simulink model "OBCSystem"  (R2025b)
settings: Solver=FixedStepAuto  StartTime=0.0  StopTime=100e-3  RelTol=1e-3  EnableMultiTasking=on
PreLoadFcn:
  | %% Load OBCSystem initialization parameters
  | initScriptPath = fullfile(fileparts(which('OBCSystem')), '..', 'SupportFiles', 'Scripts', 'OBCSystem_init.m');
  | if isfile(initScriptPath)
  |     evalin('base', fileread(initScriptPath));
  | else
  |     warning('OBCSystem:initNotFound', 'OBCSystem_init.m not found at: %s', initScriptPath);
  | end
InitFcn:
  | mode = str2double(get_param('OBCSystem/System/SimulationMode','value'));
  | enableLogging = str2double(get_param('OBCSystem/System/On-Board Charger/HIL/EnableHighResLogging','value'));
  | 
  | % If the charger runs on the FPGA AND high-resolution logging is enabled,
  | % uncomment interrupt setup. Comment otherwise
  | if ((mode == 2) && (enableLogging == 1))
  |     set_param('OBCSystem/Interrupt Setup','Commented','off');
  | else
  |     set_param('OBCSystem/Interrupt Setup','Commented','on');
  | end
  | 
  | % If DMA streaming is enambled and simulation time exceeds 30s, then throw an error
  | maxStopTime = 30;   % seconds
  | stopTimeStr = get_param(bdroot, 'StopTime');
  | stopTimeVal = str2double(stopTimeStr);
  | 
  | if enableLogging && stopTimeVal > maxStopTime
  |     error('DMA streaming is enabled, but StopTime = %.3f s exceeds the allowed %.3f s.', ...
  |           stopTimeVal, maxStopTime);
  | end
undefined symbols (not defined in the file): DAB, DAB_CCCV_Ki, DAB_CCCV_Kp, DAB_CCCV_Kt, DAB_Charging, DAB_CurrentReference, DAB_DCOffset, DAB_PhaseShift_LowerSat, DAB_PhaseShift_UpperSat, DAB_PhaseShiftInit, DAB_PhaseToDeg, DAB_PID_Kd, DAB_PID_Ki, DAB_PID_Kp, DAB_PID_LowerSat, DAB_PID_N, DAB_PID_UpperSat, Fourier_class, FPGA, FrameSize, getfullname, grid, Instr_EffGain, Instr_PinGain, Instr_PoutGain, Instr_pUtoDeg, Instr_RippleGain, Instr_SoCGain, IO334, Ki_current, Ki_voltage, Kp_current, Kp_voltage, MIL_or_HIL, OBC_template1, OpenLoopDuty, OpenLoopEnable, PCIe_RT, PFC_Current_Kb, PFC_Current_LowerSat, PFC_Current_UpperSat, PFC_Sat_DC_Lower, PFC_Sat_DC_Upper, PFC_Sat_iL_Lower, PFC_Sat_iL_Upper, PFC_Sat_Pwr_Lower, PFC_Sat_Pwr_Upper, PFC_Voltage_Kb, PFC_Voltage_LowerSat, PFC_Voltage_UpperSat, Rblock, Real, Time, totemPole, ts_CPU, ts_FPGA_clk, ts_FPGA_mdl, VectorSize
libraries: nesl_utility x27, fl_lib x24, speedgoatlib_hdlCoder_IO3xx x20, ee_lib x12, simulink x4, eeGeneralControl x4, slpidlib x3, pwm_cpulib x2, batteryecm_lib x2, slrealtimeloglib x2, pwm_fpgalib x2, speedgoatlib_interrupt x1
(part 2 of 4)

== system OBCSystem/User Interface/Instrumentation/Fourier1 ==
  In : Inport
  Fourier Analysis : eeGeneralControl/Fourier Analysis  f=50  n=2  M0=Fourier_class([0 0]).objParamMappingDerived.NewDerivedParam.M0  Ph0=Fourier_class([0 0]).objParamMappingDerived.NewDerivedParam.Ph0  BufferSize=8192  Ts=ts_CPU
  Gain : Gain  Gain=180/pi
  Mag : Outport  VectorParamsAs1DForOutWhenUnconnected=off
  Phase : Outport  Port=2  VectorParamsAs1DForOutWhenUnconnected=off
  wires:
  Gain/1 -> Phase/1
  Fourier Analysis/2 -> Gain/1
  Fourier Analysis/1 -> Mag/1
  In/1 -> Fourier Analysis/1

== system OBCSystem/User Interface/Instrumentation/Mean1 ==
  In : Inport
  Moving Average : eeGeneralControl/Moving Average  VariantControl=Variant1  LabelModeActiveChoice=Discrete  f=Instr_MeanFreq  x0=0  BufferSize=8192  Ts=ts_CPU
  Mean : Outport  VectorParamsAs1DForOutWhenUnconnected=off
  wires:
  Moving Average/1 -> Mean/1
  In/1 -> Moving Average/1

== system OBCSystem/User Interface/Instrumentation/Mean2 ==
  In : Inport
  Moving Average : eeGeneralControl/Moving Average  VariantControl=Variant1  LabelModeActiveChoice=Discrete  f=Instr_MeanFreq  x0=0  BufferSize=8192  Ts=ts_CPU
  Mean : Outport  VectorParamsAs1DForOutWhenUnconnected=off
  wires:
  Moving Average/1 -> Mean/1
  In/1 -> Moving Average/1

== system OBCSystem/User Interface/Instrumentation/THD ==
  In : Inport
  Gain : Gain  Gain=1/100  SampleTime=ts_CPU
  Total Harmonic Distortion : eeTotalHarmonicDistorsion/Total Harmonic Distortion  f=50  Ts=ts_CPU
  THD : Outport  VectorParamsAs1DForOutWhenUnconnected=off
  wires:
  Gain/1 -> THD/1
  In/1 -> Total Harmonic Distortion/1
  Total Harmonic Distortion/1 -> Gain/1

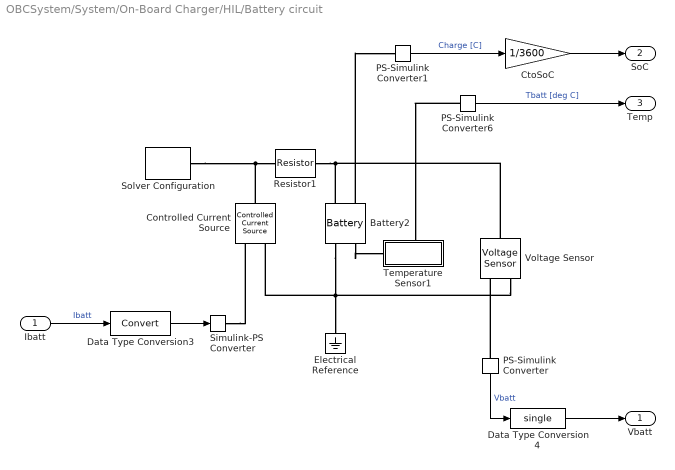
== system OBCSystem/System/On-Board Charger/HIL/Battery circuit ==
  Ibatt : Inport
  Battery2 : batteryecm_lib/Battery  Vnom=Battery_Vnom V  prm_dir=simscape.enum.battery.prm_dir.disabled  R1_dis=2 Ohm  R1_ch=2 Ohm  R1=Battery_R1 Ohm  prm_AH=simscape.enum.battery.prm_AH.finite  AH=Battery_AH A*hr  V1=Battery_V1 V  AH1=Battery_AH1 A*hr  prm_R2=simscape.enum.battery.prm_R2.disabled  R2=2000 Ohm  Tmeas=298.15 K  charge_measurement_port=simscape.enum.battery.enable.yes  prm_dyn=simscape.enum.battery.prm_dyn.off  Rp1=0.005 Ohm  tau1=30 s  Rp2=0.005 Ohm  tau2=30 s  Rp3=0.005 Ohm  tau3=30 s  Rp4=0.005 Ohm  tau4=30 s  Rp5=0.005 Ohm  tau5=30 s  prm_fade=simscape.enum.battery.prm_fade.disabled  N_fade=100  AH_fade=45 A*hr  R1_fade=2.02 Ohm  R1_ch_fade=2.02 Ohm  V1_fade=10.35 V  prm_age=simscape.enum.battery.prm_age.disabled  prm_age_OCV=simscape.enum.battery.prm_age_OCV.OCV  OCV_age=0.9  SOC_age=60  Tmeas_age=298.15 K  delta_time_age_vec=[0] d  temperature_age_vec=[273] K  OCV_scaling_age=2.2134e6  OCV_offset_age=1.632e6  temp_exp_age=0.515833569 V  t_exp_age=0.75  Vnom_T2=12 V  R1_T2=2.2 Ohm  R1_T2_dis=2.2 Ohm  R1_T2_ch=2.2 Ohm  V1_T2=11.4 V  R2_T2=2200 Ohm  Rp1_T2=0.005 Ohm  tau1_T2=30 s  Rp2_T2=0.005 Ohm  tau2_T2=30 s  Rp3_T2=0.005 Ohm  tau3_T2=30 s  Rp4_T2=0.005 Ohm  tau4_T2=30 s  Rp5_T2=0.005 Ohm  tau5_T2=30 s  Tmeas2=273.15 K  thermal_port=simscape.enum.thermaleffects.model  thermal_mass=Battery_ThermalMass J/K  i_specify=off  i_priority=None  i=0 A  i_nominal_specify=off  i_nominal_value=1  i_nominal_unit=A  v_specify=off  v_priority=High  v=380 V  v_nominal_specify=off  v_nominal_value=1  v_nominal_unit=V  charge_specify=on  charge_priority=High  charge=Battery_InitCharge A*hr  charge_nominal_specify=off  charge_nominal_value=1  charge_nominal_unit=A*hr  num_cycles_specify=off  num_cycles_priority=High  num_cycles=0  num_cycles_nominal_specify=off  num_cycles_nominal_value=1  num_cycles_nominal_unit=1  temperature_specify=off  temperature_priority=High  temperature=298.15 K  temperature_nominal_specify=off  temperature_nominal_value=1  temperature_nominal_unit=K
      settings: InternalSimscapePortConfiguration="{\"Bottom\":[],\"Left\":[{\"id\":\"p\",\"label\":\"+\",\"type\":\"foundation.electrical.electrical\"},{\"id\":\"q\",\"label\":\"q\",\"type\":\"output\"}],\"Right\":[{\"id\":\"n\",\"label\":\"-\",\"type\":\"foundation.electrical.electrical\"},{\"id\":\"H\",\"label\":\"H\",\"type\":\"foundation.thermal.thermal\"}],\"Top\":[]}"
  Controlled Current Source : fl_lib/Electrical/Electrical Sources/Controlled Current Source
  CtoSoC : Gain  Gain=1/3600
  Data Type Conversion3 : DataTypeConversion  SaturateOnIntegerOverflow=off  RndMeth=Floor
  Data Type Conversion4 : DataTypeConversion  OutDataTypeStr=single  SaturateOnIntegerOverflow=off  RndMeth=Floor
  Electrical Reference : fl_lib/Electrical/Electrical Elements/Electrical Reference
  PS-Simulink Converter : nesl_utility/PS-Simulink Converter  PhysicalDomain=network_engine_domain  SubClassName=ps_output  LeftPortType=input  RightPortType=output  PseudoPeriodic=off  Frequencies=[]  VectorFormat=inherit  Unit=inherit  AffineConversion=off
  PS-Simulink Converter1 : nesl_utility/PS-Simulink Converter  PhysicalDomain=network_engine_domain  SubClassName=ps_output  LeftPortType=input  RightPortType=output  PseudoPeriodic=off  Frequencies=[]  VectorFormat=inherit  Unit=inherit  AffineConversion=off
  PS-Simulink Converter6 : nesl_utility/PS-Simulink Converter  PhysicalDomain=network_engine_domain  SubClassName=ps_output  LeftPortType=input  RightPortType=output  PseudoPeriodic=off  Frequencies=[]  VectorFormat=inherit  Unit=inherit  AffineConversion=off
  Resistor1 : fl_lib/Electrical/Electrical Elements/Resistor  R=0.1 Ohm  i_specify=off  i_priority=None  i=0 A  i_nominal_specify=off  i_nominal_value=1  i_nominal_unit=A  v_specify=off  v_priority=None  v=0 V  v_nominal_specify=off  v_nominal_value=1  v_nominal_unit=V
  Simulink-PS Converter : nesl_utility/Simulink-PS Converter  PhysicalDomain=network_engine_domain  SubClassName=ps_input  LeftPortType=input  RightPortType=output  PseudoPeriodic=off  Frequencies=[]  NoiseDistribution=none  NoiseParameters=[]  Unit=1  AffineConversion=off  FilteringAndDerivatives=provide  SimscapeFilterOrder=1  InputFilterTimeConstant=0.001  UdotUserProvided=0
  Solver Configuration : nesl_utility/Solver Configuration  PhysicalDomain=network_engine_domain  SubClassName=solver  LeftPortType=input  RightPortType=generic  Tones=[]  Harmonics=[]  SimulateNoise=off  Profile=off  UseLocalSampling=off  EnableSwitchedLinearOptims=on  FrequencyDomain=off  UseCCode=off  RelTol=0.001  AbsTol=0.001  MinStep=1e-09  ToWorkspace=off  RevertToSquareIcSolve=off  NumHomotopyIterations=100  PhasorMode=off  PhasorModeNumHarmonics=1  ConsistencySolver=NEWTON_XTOL_AFTER_FTOL  IndexReductionMethod=DerivativeReplacement  DoDC=off  ResidualTolerance=1e-09  ConsistencyTolSource=GLOBAL  ConsistencyAbsTol=0.001  ConsistencyRelTol=0.001  ConsistencyTolFactor=0.001  UseLocalSolver=on  LocalSolverChoice=NE_BACKWARD_EULER_ADVANCER  ResolveIndetEquations=on  FunctionEvalNumThread=1  LocalSolverSampleTime=5e-5  DoFixedCost=on  MaxNonlinIter=3  MaxModeIter=2  ComputeImpulses=off  ImpulseIterations=2  LinearAlgebra=auto  LinearAlgebraNumThread=0  EquationFormulation=NE_TIME_EF  DelaysMemoryBudget=1024  AutomaticFiltering=on  FilteringTimeConstant=0.001  PartitionStorageMethod=AS_NEEDED  PartitionMemoryBudget=1024  PartitionMethod=ROBUST  MultibodyUseLocalSolver=off  MultibodyLocalSolverChoice=ODE1  MultibodyLocalSolverSampleTime=0.001
  Temperature Sensor1 : Subsystem
      settings: PortSchema="{\"entries\":[{\"content\":{\"sides\":[{\"content\":{\"connectorIds\":[\"LConn1\"]},\"type\":\"ConnectorPlacement.EquallySpacedRectSide\",\"uuid\":\"ed56c3af-3423-4ba9-9558-54e91d6a43d9\"},{\"content\":{\"side\":\"RIGHT\"},\"type\":\"ConnectorPlacement.EquallySpacedRectSide\",\"uuid\":\"9f5709b7-2572-4890-9020-500e0d1722b1\"},{\"content\":{\"connectorIds\":[\"LConn2\"],\"side\":\"TOP\"},\"type\":\"ConnectorPlacement.EquallySpacedRectSide\",\"uuid\":\"64165555-65dc-4e1f-8e23-cd71f1c59f36\"}]},\"type\":\"ConnectorPlacement.EquallySpacedConnector\",\"uuid\":\"8bb26fd1-535d-4a0d-a366-f45db75374c2\"}],\"packageUris\":[\"http://schema.mathworks.com/mf0/Connector/R2020b\"],\"version\":\"1.0\"}"
  Voltage Sensor : fl_lib/Electrical/Electrical Sensors/Voltage Sensor
  Vbatt : Outport
  SoC : Outport  Port=2
  Temp : Outport  Port=3
  wires:
  PS-Simulink Converter1/1 -> CtoSoC/1  "Charge [C]"
  Ibatt/1 -> Data Type Conversion3/1  "Ibatt"
  Data Type Conversion4/1 -> Vbatt/1
  PS-Simulink Converter/1 -> Data Type Conversion4/1  "Vbatt"
  CtoSoC/1 -> SoC/1
  Data Type Conversion3/1 -> Simulink-PS Converter/1
  PS-Simulink Converter6/1 -> Temp/1  "Tbatt [deg C]"
  connections:
  Controlled Current Source/RConn2 -- Battery2/RConn1 -- Electrical Reference/LConn1 -- Voltage Sensor/RConn2
  PS-Simulink Converter/LConn1 -- Voltage Sensor/RConn1
  Simulink-PS Converter/RConn1 -- Controlled Current Source/RConn1
  Battery2/RConn2 -- Temperature Sensor1/LConn1
  Voltage Sensor/LConn1 -- Battery2/LConn1 -- Resistor1/RConn1
  Battery2/LConn2 -- PS-Simulink Converter1/LConn1
  PS-Simulink Converter6/LConn1 -- Temperature Sensor1/LConn2
  Solver Configuration/RConn1 -- Resistor1/LConn1 -- Controlled Current Source/LConn1

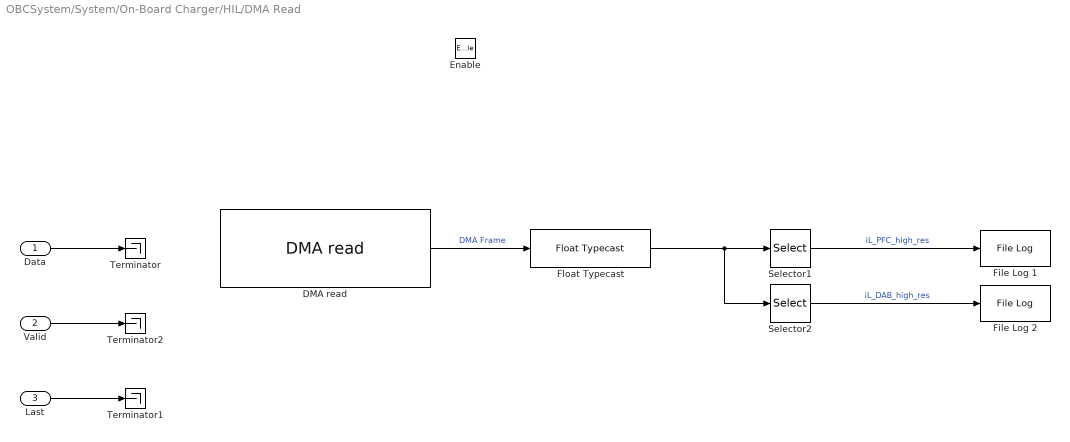
== system OBCSystem/System/On-Board Charger/HIL/DMA Read ==
  Data : Inport
  Valid : Inport  Port=2
  Last : Inport  Port=3
  Enable : EnablePort
  DMA read : speedgoatlib_hdlCoder_IO3xx_user/DMA read  module_id=1  dma_transfer_size=FrameSize  dma_polling=off  sample_time=ts_CPU  word_count=off
      settings: SourceProductName=IO3xx User
  File Log 1 : slrealtimeloglib/File Log  decimation=1  inputProcessing=Columns as channels (frame based)
  File Log 2 : slrealtimeloglib/File Log  decimation=1  inputProcessing=Columns as channels (frame based)
  Float Typecast : FloatTypecast
  Selector1 : Selector  IndexOptions=Index vector (dialog)  Indices=1:VectorSize:FrameSize  OutputSizes=1
  Selector2 : Selector  IndexOptions=Index vector (dialog)  Indices=2:VectorSize:FrameSize  OutputSizes=1
  Terminator : Terminator
  Terminator1 : Terminator
  Terminator2 : Terminator
  wires:
  Data/1 -> Terminator/1
  Last/1 -> Terminator1/1
  Valid/1 -> Terminator2/1
  Selector1/1 -> File Log 1/1  "iL_PFC_high_res"
  Float Typecast/1 -> Selector2/1, Selector1/1
  DMA read/1 -> Float Typecast/1  "DMA Frame"
  Selector2/1 -> File Log 2/1  "iL_DAB_high_res"

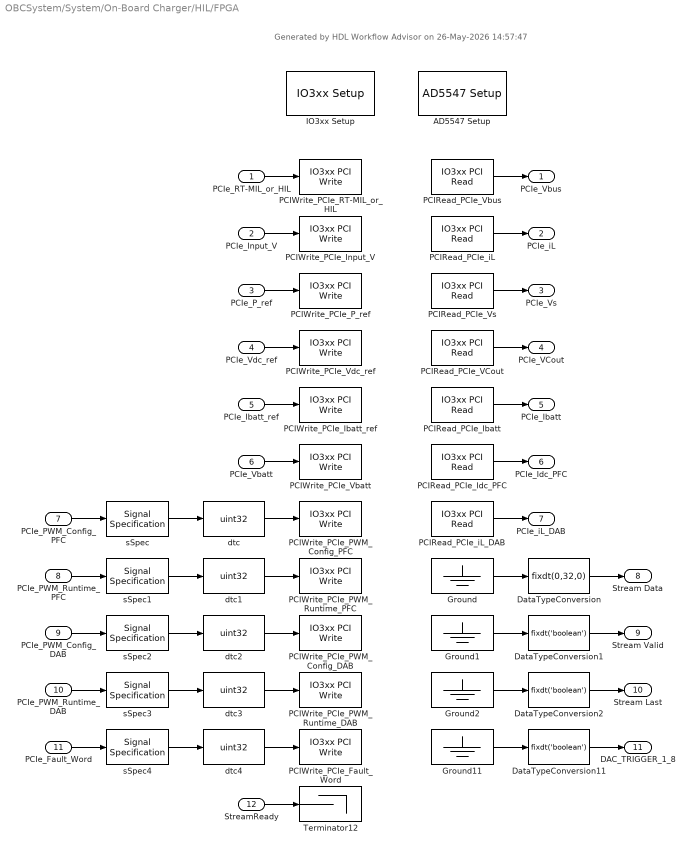
== system OBCSystem/System/On-Board Charger/HIL/FPGA ==
  note: Generated by HDL Workflow Advisor on 26-May-2026 14:57:47
  PCIe_RT-MIL_or_HIL : Inport
  PCIe_Input_V : Inport  Port=2
  PCIe_P_ref : Inport  Port=3
  PCIe_Vdc_ref : Inport  Port=4
  PCIe_Ibatt_ref : Inport  Port=5
  PCIe_Vbatt : Inport  Port=6
  PCIe_PWM_Config_PFC : Inport  Port=7
  PCIe_PWM_Runtime_PFC : Inport  Port=8
  PCIe_PWM_Config_DAB : Inport  Port=9
  PCIe_PWM_Runtime_DAB : Inport  Port=10
  PCIe_Fault_Word : Inport  Port=11
  StreamReady : Inport  Port=12
  AD5547 Setup : speedgoatlib_hdlCoder_IO3xx/AD5547 Setup  module_id=module_id  dacReset=on  dacGain_1=+/- 10.0V  dacActiv_1=on  dacInit_1=dacInit_1  dacGain_2=+/- 10.0V  dacActiv_2=on  dacInit_2=dacInit_2  dacGain_3=+/- 10.0V  dacActiv_3=on  dacInit_3=dacInit_3  dacGain_4=+/- 10.0V  dacActiv_4=on  dacInit_4=dacInit_4  dacGain_5=+/- 10.0V  dacActiv_5=on  dacInit_5=dacInit_5  dacGain_6=+/- 10.0V  dacActiv_6=on  dacInit_6=dacInit_6  dacGain_7=+/- 10.0V  dacActiv_7=on  dacInit_7=dacInit_7  dacGain_8=+/- 10.0V  dacActiv_8=on  dacInit_8=dacInit_8  dacGain_9=+/- 10.0V  dacActiv_9=off  dacInit_9=dacInit_9  dacGain_10=+/- 10.0V  dacActiv_10=off  dacInit_10=dacInit_10  dacGain_11=+/- 10.0V  dacActiv_11=off  dacInit_11=dacInit_11  dacGain_12=+/- 10.0V  dacActiv_12=off  dacInit_12=dacInit_12  dacGain_13=+/- 10.0V  dacActiv_13=off  dacInit_13=dacInit_13  dacGain_14=+/- 10.0V  dacActiv_14=off  dacInit_14=dacInit_14  dacGain_15=+/- 10.0V  dacActiv_15=off  dacInit_15=dacInit_15  dacGain_16=+/- 10.0V  dacActiv_16=off  dacInit_16=dacInit_16  dacGain_17=+/- 10.0V  dacActiv_17=off  dacInit_17=dacInit_17  dacGain_18=+/- 10.0V  dacActiv_18=off  dacInit_18=dacInit_18  dacGain_19=+/- 10.0V  dacActiv_19=off  dacInit_19=dacInit_19  dacGain_20=+/- 10.0V  dacActiv_20=off  dacInit_20=dacInit_20  dacGain_21=+/- 10.0V  dacActiv_21=off  dacInit_21=dacInit_21  dacGain_22=+/- 10.0V  dacActiv_22=off  dacInit_22=dacInit_22  dacGain_23=+/- 10.0V  dacActiv_23=off  dacInit_23=dacInit_23  dacGain_24=+/- 10.0V  dacActiv_24=off  dacInit_24=dacInit_24  dacGain_25=+/- 10.0V  dacActiv_25=off  dacInit_25=dacInit_25  dacGain_26=+/- 10.0V  dacActiv_26=off  dacInit_26=dacInit_26  dacGain_27=+/- 10.0V  dacActiv_27=off  dacInit_27=dacInit_27  dacGain_28=+/- 10.0V  dacActiv_28=off  dacInit_28=dacInit_28  dacGain_29=+/- 10.0V  dacActiv_29=off  dacInit_29=dacInit_29  dacGain_30=+/- 10.0V  dacActiv_30=off  dacInit_30=dacInit_30  dacGain_31=+/- 10.0V  dacActiv_31=off  dacInit_31=dacInit_31  dacGain_32=+/- 10.0V  dacActiv_32=off  dacInit_32=dacInit_32
  DataTypeConversion : DataTypeConversion  OutDataTypeStr=fixdt(0,32,0)  ConvertRealWorld=Stored Integer (SI)  SaturateOnIntegerOverflow=off  RndMeth=Floor
  DataTypeConversion1 : DataTypeConversion  OutDataTypeStr=fixdt('boolean')  ConvertRealWorld=Stored Integer (SI)  SaturateOnIntegerOverflow=off  RndMeth=Floor
  DataTypeConversion11 : DataTypeConversion  OutDataTypeStr=fixdt('boolean')  ConvertRealWorld=Stored Integer (SI)  SaturateOnIntegerOverflow=off  RndMeth=Floor
  DataTypeConversion2 : DataTypeConversion  OutDataTypeStr=fixdt('boolean')  ConvertRealWorld=Stored Integer (SI)  SaturateOnIntegerOverflow=off  RndMeth=Floor
  Ground{,1..2,11} (4 alike) : Ground
  IO3xx Setup : speedgoatlib_hdlCoder_IO3xx/IO3xx Setup  mdl_ss_name=OBC_template1/FPGA  board_type=IO334-325k  fpga_sync_mode=on  reset_mode=on  reset_mode_stop=on  device_id=1  module_id=module_id  pci_slot=slot  fpga_mat_file=hdl_prj\hdlsrc\OBC_template1\FPGA.mat  timestamp_mcs=05/26/26 14:55:02  timestamp=3535072706  tsreg=hex2dec('8')  bsf_file=FPGA_2605261424.mcs  mcs=0  init_reg_list=[]
  PCIRead_PCIe_Ibatt : speedgoatlib_hdlCoder_IO3xx/IO3xx PCI Read  device_id=1  module_id=module_id  board_type=IO334-325k  port_name=PCIe_Ibatt  port_offset=hex2dec('800')  port_type=single  port_dim=1  strobe=0  sample_time=ts
  PCIRead_PCIe_Idc_PFC : speedgoatlib_hdlCoder_IO3xx/IO3xx PCI Read  device_id=1  module_id=module_id  board_type=IO334-325k  port_name=PCIe_Idc_PFC  port_offset=hex2dec('108')  port_type=single  port_dim=1  strobe=0  sample_time=ts
  PCIRead_PCIe_VCout : speedgoatlib_hdlCoder_IO3xx/IO3xx PCI Read  device_id=1  module_id=module_id  board_type=IO334-325k  port_name=PCIe_VCout  port_offset=hex2dec('120')  port_type=single  port_dim=1  strobe=0  sample_time=ts
  PCIRead_PCIe_Vbus : speedgoatlib_hdlCoder_IO3xx/IO3xx PCI Read  device_id=1  module_id=module_id  board_type=IO334-325k  port_name=PCIe_Vbus  port_offset=hex2dec('110')  port_type=single  port_dim=1  strobe=0  sample_time=ts
  PCIRead_PCIe_Vs : speedgoatlib_hdlCoder_IO3xx/IO3xx PCI Read  device_id=1  module_id=module_id  board_type=IO334-325k  port_name=PCIe_Vs  port_offset=hex2dec('130')  port_type=single  port_dim=1  strobe=0  sample_time=ts
  PCIRead_PCIe_iL : speedgoatlib_hdlCoder_IO3xx/IO3xx PCI Read  device_id=1  module_id=module_id  board_type=IO334-325k  port_name=PCIe_iL  port_offset=hex2dec('114')  port_type=single  port_dim=1  strobe=0  sample_time=ts
  PCIRead_PCIe_iL_DAB : speedgoatlib_hdlCoder_IO3xx/IO3xx PCI Read  device_id=1  module_id=module_id  board_type=IO334-325k  port_name=PCIe_iL_DAB  port_offset=hex2dec('124')  port_type=single  port_dim=1  strobe=0  sample_time=ts
  PCIWrite_PCIe_Fault_Word : speedgoatlib_hdlCoder_IO3xx/IO3xx PCI Write  device_id=1  module_id=module_id  board_type=IO334-325k  port_name=PCIe_Fault_Word  port_offset=hex2dec('10C')  port_type=uint32  port_dim=1  strobe=0  sample_time=ts
  PCIWrite_PCIe_Ibatt_ref : speedgoatlib_hdlCoder_IO3xx/IO3xx PCI Write  device_id=1  module_id=module_id  board_type=IO334-325k  port_name=PCIe_Ibatt_ref  port_offset=hex2dec('100')  port_type=single  port_dim=1  strobe=0  sample_time=ts
  PCIWrite_PCIe_Input_V : speedgoatlib_hdlCoder_IO3xx/IO3xx PCI Write  device_id=1  module_id=module_id  board_type=IO334-325k  port_name=PCIe_Input_V  port_offset=hex2dec('12C')  port_type=single  port_dim=1  strobe=0  sample_time=ts
  PCIWrite_PCIe_PWM_Config_DAB : speedgoatlib_hdlCoder_IO3xx/IO3xx PCI Write  device_id=1  module_id=module_id  board_type=IO334-325k  port_name=PCIe_PWM_Config_DAB  port_offset=hex2dec('200')  port_type=uint32  port_dim=32  strobe=hex2dec('280')  sample_time=ts
  PCIWrite_PCIe_PWM_Config_PFC : speedgoatlib_hdlCoder_IO3xx/IO3xx PCI Write  device_id=1  module_id=module_id  board_type=IO334-325k  port_name=PCIe_PWM_Config_PFC  port_offset=hex2dec('140')  port_type=uint32  port_dim=16  strobe=hex2dec('180')  sample_time=ts
  PCIWrite_PCIe_PWM_Runtime_DAB : speedgoatlib_hdlCoder_IO3xx/IO3xx PCI Write  device_id=1  module_id=module_id  board_type=IO334-325k  port_name=PCIe_PWM_Runtime_DAB  port_offset=hex2dec('2C0')  port_type=uint32  port_dim=10  strobe=hex2dec('300')  sample_time=ts
  PCIWrite_PCIe_PWM_Runtime_PFC : speedgoatlib_hdlCoder_IO3xx/IO3xx PCI Write  device_id=1  module_id=module_id  board_type=IO334-325k  port_name=PCIe_PWM_Runtime_PFC  port_offset=hex2dec('1A0')  port_type=uint32  port_dim=5  strobe=hex2dec('1C0')  sample_time=ts
  PCIWrite_PCIe_P_ref : speedgoatlib_hdlCoder_IO3xx/IO3xx PCI Write  device_id=1  module_id=module_id  board_type=IO334-325k  port_name=PCIe_P_ref  port_offset=hex2dec('118')  port_type=single  port_dim=1  strobe=0  sample_time=ts
  PCIWrite_PCIe_RT-MIL_or_HIL : speedgoatlib_hdlCoder_IO3xx/IO3xx PCI Write  device_id=1  module_id=module_id  board_type=IO334-325k  port_name=PCIe_RT-MIL_or_HIL  port_offset=hex2dec('128')  port_type=single  port_dim=1  strobe=0  sample_time=ts
  PCIWrite_PCIe_Vbatt : speedgoatlib_hdlCoder_IO3xx/IO3xx PCI Write  device_id=1  module_id=module_id  board_type=IO334-325k  port_name=PCIe_Vbatt  port_offset=hex2dec('104')  port_type=single  port_dim=1  strobe=0  sample_time=ts
  PCIWrite_PCIe_Vdc_ref : speedgoatlib_hdlCoder_IO3xx/IO3xx PCI Write  device_id=1  module_id=module_id  board_type=IO334-325k  port_name=PCIe_Vdc_ref  port_offset=hex2dec('11C')  port_type=single  port_dim=1  strobe=0  sample_time=ts
  Terminator12 : Terminator
  dtc{,1..4} (5 alike) : DataTypeConversion  OutDataTypeStr=uint32  ConvertRealWorld=Stored Integer (SI)  SaturateOnIntegerOverflow=off
  sSpec{,1..4} (5 alike) : SignalSpecification  OutDataTypeStr=fixdt(0,32,0)
  PCIe_Vbus : Outport
  PCIe_iL : Outport  Port=2
  PCIe_Vs : Outport  Port=3
  PCIe_VCout : Outport  Port=4
  PCIe_Ibatt : Outport  Port=5
  PCIe_Idc_PFC : Outport  Port=6
  PCIe_iL_DAB : Outport  Port=7
  Stream Data : Outport  Port=8
  Stream Valid : Outport  Port=9
  Stream Last : Outport  Port=10
  DAC_TRIGGER_1_8 : Outport  Port=11
  wires:
  PCIe_RT-MIL_or_HIL/1 -> PCIWrite_PCIe_RT-MIL_or_HIL/1
  PCIe_Input_V/1 -> PCIWrite_PCIe_Input_V/1
  PCIe_P_ref/1 -> PCIWrite_PCIe_P_ref/1
  PCIe_Vdc_ref/1 -> PCIWrite_PCIe_Vdc_ref/1
  PCIe_Ibatt_ref/1 -> PCIWrite_PCIe_Ibatt_ref/1
  PCIe_Vbatt/1 -> PCIWrite_PCIe_Vbatt/1
  PCIe_PWM_Config_PFC/1 -> sSpec/1
  sSpec/1 -> dtc/1
  dtc/1 -> PCIWrite_PCIe_PWM_Config_PFC/1
  PCIe_PWM_Runtime_PFC/1 -> sSpec1/1
  sSpec1/1 -> dtc1/1
  dtc1/1 -> PCIWrite_PCIe_PWM_Runtime_PFC/1
  PCIe_PWM_Config_DAB/1 -> sSpec2/1
  sSpec2/1 -> dtc2/1
  dtc2/1 -> PCIWrite_PCIe_PWM_Config_DAB/1
  PCIe_PWM_Runtime_DAB/1 -> sSpec3/1
  sSpec3/1 -> dtc3/1
  dtc3/1 -> PCIWrite_PCIe_PWM_Runtime_DAB/1
  PCIe_Fault_Word/1 -> sSpec4/1
  sSpec4/1 -> dtc4/1
  dtc4/1 -> PCIWrite_PCIe_Fault_Word/1
  PCIRead_PCIe_Vbus/1 -> PCIe_Vbus/1
  PCIRead_PCIe_iL/1 -> PCIe_iL/1
  PCIRead_PCIe_Vs/1 -> PCIe_Vs/1
  PCIRead_PCIe_VCout/1 -> PCIe_VCout/1
  PCIRead_PCIe_Ibatt/1 -> PCIe_Ibatt/1
  PCIRead_PCIe_Idc_PFC/1 -> PCIe_Idc_PFC/1
  PCIRead_PCIe_iL_DAB/1 -> PCIe_iL_DAB/1
  StreamReady/1 -> Terminator12/1
  DataTypeConversion/1 -> Stream Data/1
  Ground/1 -> DataTypeConversion/1
  DataTypeConversion1/1 -> Stream Valid/1
  Ground1/1 -> DataTypeConversion1/1
  DataTypeConversion2/1 -> Stream Last/1
  Ground2/1 -> DataTypeConversion2/1
  DataTypeConversion11/1 -> DAC_TRIGGER_1_8/1
  Ground11/1 -> DataTypeConversion11/1

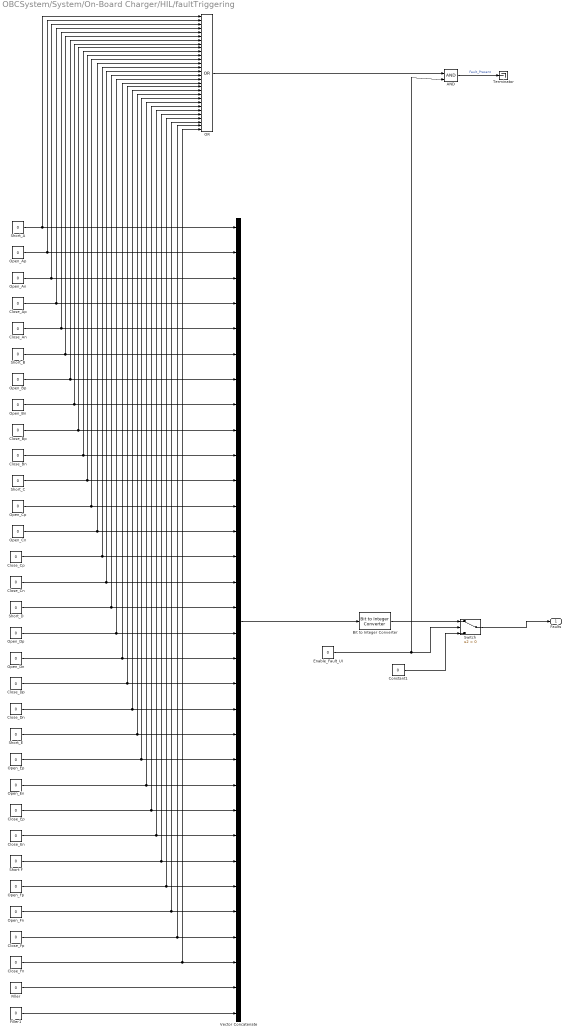
== system OBCSystem/System/On-Board Charger/HIL/faultTriggering ==
  AND : Logic  IconShape=distinctive  AllPortsSameDT=off  OutDataTypeStr=boolean
  Bit to Integer Converter : simulink/Logic and Bit Operations/Bit to Integer Converter  nbits=32  bitOrder=LSB first  signedOutputValues=Unsigned  outDtype=uint32  outDtypeSigned=Inherit via internal rule
  Close_An : Constant  Value=0  OutDataTypeStr=boolean  SampleTime=-1
  Close_Ap : Constant  Value=0  OutDataTypeStr=boolean  SampleTime=-1
  Close_Bn : Constant  Value=0  OutDataTypeStr=boolean  SampleTime=-1
  Close_Bp : Constant  Value=0  OutDataTypeStr=boolean  SampleTime=-1
  Close_Cn : Constant  Value=0  OutDataTypeStr=boolean  SampleTime=-1
  Close_Cp : Constant  Value=0  OutDataTypeStr=boolean  SampleTime=-1
  Close_Dn : Constant  Value=0  OutDataTypeStr=boolean  SampleTime=-1
  Close_Dp : Constant  Value=0  OutDataTypeStr=boolean  SampleTime=-1
  Close_En : Constant  Value=0  OutDataTypeStr=boolean  SampleTime=-1
  Close_Ep : Constant  Value=0  OutDataTypeStr=boolean  SampleTime=-1
  Close_Fn : Constant  Value=0  OutDataTypeStr=boolean  SampleTime=-1
  Close_Fp : Constant  Value=0  OutDataTypeStr=boolean  SampleTime=-1
  Constant1 : Constant  Value=0  OutDataTypeStr=uint32  SampleTime=ts_CPU
  Enable_Fault_UI : Constant  Value=0  OutDataTypeStr=boolean  SampleTime=ts_CPU
  Filler : Constant  Value=0  OutDataTypeStr=boolean  SampleTime=-1
  Filler1 : Constant  Value=0  OutDataTypeStr=boolean  SampleTime=-1
  OR : Logic  Operator=OR  Inputs=30  IconShape=distinctive  AllPortsSameDT=off  OutDataTypeStr=boolean
  Open_An : Constant  Value=0  OutDataTypeStr=boolean  SampleTime=-1
  Open_Ap : Constant  Value=0  OutDataTypeStr=boolean  SampleTime=-1
  Open_Bn : Constant  Value=0  OutDataTypeStr=boolean  SampleTime=-1
  Open_Bp : Constant  Value=0  OutDataTypeStr=boolean  SampleTime=-1
  Open_Cn : Constant  Value=0  OutDataTypeStr=boolean  SampleTime=-1
  Open_Cp : Constant  Value=0  OutDataTypeStr=boolean  SampleTime=-1
  Open_Dn : Constant  Value=0  OutDataTypeStr=boolean  SampleTime=-1
  Open_Dp : Constant  Value=0  OutDataTypeStr=boolean  SampleTime=-1
  Open_En : Constant  Value=0  OutDataTypeStr=boolean  SampleTime=-1
  Open_Ep : Constant  Value=0  OutDataTypeStr=boolean  SampleTime=-1
  Open_Fn : Constant  Value=0  OutDataTypeStr=boolean  SampleTime=-1
  Open_Fp : Constant  Value=0  OutDataTypeStr=boolean  SampleTime=-1
  Short F : Constant  Value=0  OutDataTypeStr=boolean  SampleTime=ts_CPU
  Short_A : Constant  Value=0  OutDataTypeStr=boolean  SampleTime=ts_CPU
  Short_B : Constant  Value=0  OutDataTypeStr=boolean  SampleTime=-1
  Short_C : Constant  Value=0  OutDataTypeStr=boolean  SampleTime=-1
  Short_D : Constant  Value=0  OutDataTypeStr=boolean  SampleTime=-1
  Short_E : Constant  Value=0  OutDataTypeStr=boolean  SampleTime=-1
  Switch : Switch  Criteria=u2 > Threshold  SaturateOnIntegerOverflow=off  InputSameDT=off
  Terminator : Terminator
  Vector Concatenate : Concatenate  NumInputs=32
  Faults : Outport
  wires:
  Open_Cp/1 -> Vector Concatenate/12, OR/12
  Close_Bp/1 -> Vector Concatenate/9, OR/9
  Short_A/1 -> Vector Concatenate/1, OR/1
  Open_Bn/1 -> Vector Concatenate/8, OR/8
  Open_Ap/1 -> Vector Concatenate/2, OR/2
  Open_An/1 -> Vector Concatenate/3, OR/3
  Close_Ap/1 -> Vector Concatenate/4, OR/4
  Close_An/1 -> Vector Concatenate/5, OR/5
  Short_B/1 -> Vector Concatenate/6, OR/6
  Filler/1 -> Vector Concatenate/31
  Short_C/1 -> Vector Concatenate/11, OR/11
  Close_Bn/1 -> Vector Concatenate/10, OR/10
  Open_Bp/1 -> Vector Concatenate/7, OR/7
  Short_D/1 -> Vector Concatenate/16, OR/16
  Open_Cn/1 -> Vector Concatenate/13, OR/13
  Open_Dn/1 -> Vector Concatenate/18, OR/18
  Open_Dp/1 -> Vector Concatenate/17, OR/17
  Close_Cn/1 -> Vector Concatenate/15, OR/15
  Close_Cp/1 -> Vector Concatenate/14, OR/14
  Close_Ep/1 -> OR/24, Vector Concatenate/24
  Open_En/1 -> OR/23, Vector Concatenate/23
  Short F/1 -> OR/26, Vector Concatenate/26
  Close_En/1 -> OR/25, Vector Concatenate/25
  Open_Ep/1 -> OR/22, Vector Concatenate/22
  Short_E/1 -> OR/21, Vector Concatenate/21
  Open_Fp/1 -> OR/27, Vector Concatenate/27
  Enable_Fault_UI/1 -> AND/2, Switch/2
  Vector Concatenate/1 -> Bit to Integer Converter/1
  Switch/1 -> Faults/1
  Bit to Integer Converter/1 -> Switch/1
  Constant1/1 -> Switch/3
  OR/1 -> AND/1
  AND/1 -> Terminator/1  "Fault_Present"
  Filler1/1 -> Vector Concatenate/32
  Close_Dp/1 -> OR/19, Vector Concatenate/19
  Close_Dn/1 -> OR/20, Vector Concatenate/20
  Open_Fn/1 -> OR/28, Vector Concatenate/28
  Close_Fp/1 -> OR/29, Vector Concatenate/29
  Close_Fn/1 -> OR/30, Vector Concatenate/30

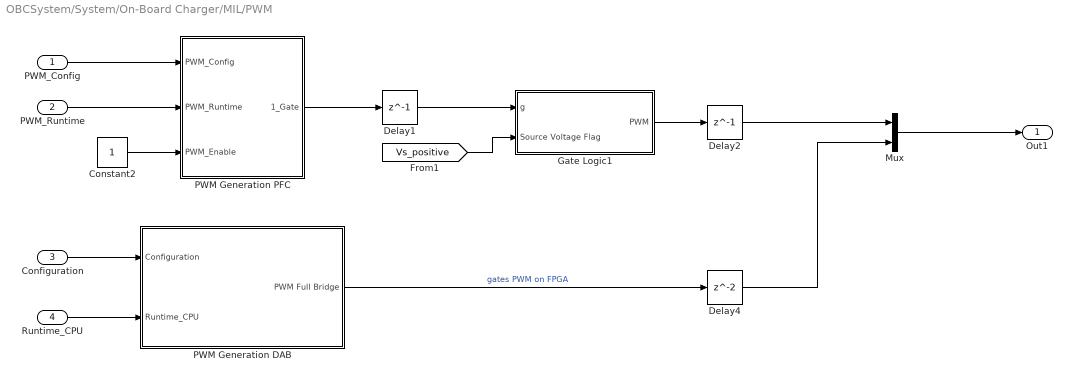
== system OBCSystem/System/On-Board Charger/MIL/PWM ==
  PWM_Config : Inport
  PWM_Runtime : Inport  Port=2
  Configuration : Inport  Port=3
  Runtime_CPU : Inport  Port=4
  Constant2 : Constant  OutDataTypeStr=boolean  SampleTime=ts_FPGA_mdl
  Delay1 : Delay  DelayLength=1
  Delay2 : Delay  DelayLength=1
  Delay4 : Delay
  Gate Logic1 : Subsystem
  Mux : Mux  Inputs=2
  "PWM Generation DAB " : Subsystem
  PWM Generation PFC : Subsystem
  Out1 : Outport
  wires:
  Gate Logic1/1(PWM) -> Delay2/1
  Delay4/1 -> Mux/2
  Mux/1 -> Out1/1
  [Vs_positive] -> Gate Logic1/2(Source Voltage Flag)
  PWM Generation PFC/1(1_Gate) -> Delay1/1
  Constant2/1 -> PWM Generation PFC/3(PWM_Enable)
  "PWM Generation DAB "/1(PWM Full Bridge) -> Delay4/1  "gates PWM on FPGA"
  Delay2/1 -> Mux/1
  Delay1/1 -> Gate Logic1/1(g)
  Configuration/1 -> "PWM Generation DAB "/1(Configuration)
  PWM_Config/1 -> PWM Generation PFC/1(PWM_Config)
  PWM_Runtime/1 -> PWM Generation PFC/2(PWM_Runtime)
  Runtime_CPU/1 -> "PWM Generation DAB "/2(Runtime_CPU)
